simulink library "Lib_NM_NewtonRaphsonSolver_TMATS"  (Simulink 8.5)
settings: Solver=ode45  StartTime=0.0  StopTime=10.0  RelTol=1e-3
Description:
  | Thomas Modules
settings Model: Creator=jwchapm2  LastModifiedBy=jwchapm2

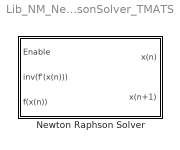
== system Lib_NM_NewtonRaphsonSolver_TMATS ==
  Newton Raphson Solver : Subsystem  TreatAsAtomicUnit=on  mask(T-MATS: Newton Raphson Solver Library Block){NR_IC_M=[1; 2; 3], NR_dx_Lim_M=5, NR_Mx_Lim_M=100000, NR_Mn_Lim_M=0.000001, BlkNm_M=double(gcb)}
      mask prompts: NR_IC_M "NR_IC_M - Initial Conditions of Newton Raphson (mx1)"; NR_dx_Lim_M "NR_dx_Lim_M - Newton Raphson step size limit (%) (1x1)"; NR_Mx_Lim_M "NR_Mx_Lim_M - Max limit (1x1 or mx1)"; NR_Mn_Lim_M "NR_Mn_Lim_M - Min Limit (1x1 or mx1)"; BlkNm_M "BlkNm_M - Block Name"
      mask help:
      | Newton Raphson Solver:
      |
      | x(n+1) = x(n) - inverse(f'(x(n)))*f(x(n))
      |
      | Note:
      | inverse(f'(x(n))) is an m x m matrix and f(x(n)) is an m x 1 matrix
      | where m is the length of the initial conditions matrix and number of system independents.
      mask init:
      | if isequal(size(NR_Mx_Lim_M),size(NR_IC_M))
      | elseif isequal(size(NR_Mx_Lim_M),size(1))
      | else
      |     warning('NR_Mx_Lim_M must be the same size as NR_IC_M or a constant')
      | end
      | 
      | if isequal(size(NR_Mn_Lim_M),size(NR_IC_M))
      | elseif isequal(size(NR_Mn_Lim_M),size(1))
      | else
      |     warning('NR_Mn_Lim_M must be the same size as NR_IC_M or a constant')
      | end
      mask Help: web(which('NumMthd_TMATS_NRS.html'),'-helpbrowser')

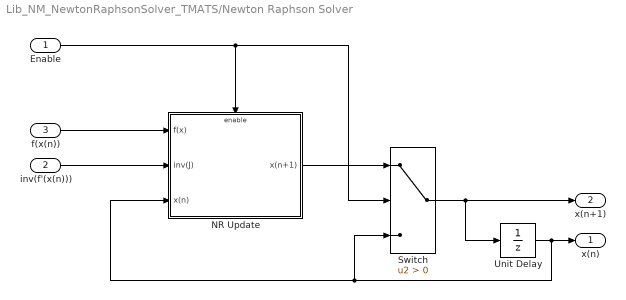
== system Lib_NM_NewtonRaphsonSolver_TMATS/Newton Raphson Solver ==
  Enable : Inport  PortDimensions=1
  inv(f'(x(n))) : Inport  Port=2  PortDimensions=[length(NR_IC_M),length(NR_IC_M)]
  f(x(n)) : Inport  Port=3  PortDimensions=length(NR_IC_M)
  NR Update : Subsystem
  Switch : Switch  Criteria=u2 > Threshold
  Unit Delay : UnitDelay  InitialCondition=NR_IC_M  SampleTime=-1
  x(n) : Outport  PortDimensions=length(NR_IC_M)
  x(n+1) : Outport  Port=2  PortDimensions=length(NR_IC_M)
  wires:
  Unit Delay/1 -> x(n)/1, Switch/3, NR Update/3(x(n))
  Enable/1 -> Switch/2, NR Update/Enable
  Switch/1 -> Unit Delay/1, x(n+1)/1
  f(x(n))/1 -> NR Update/1(f(x))
  inv(f'(x(n)))/1 -> NR Update/2(inv(J))
  NR Update/1(x(n+1)) -> Switch/1

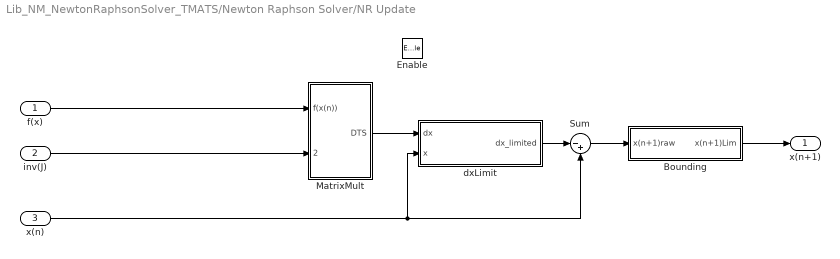
== system Lib_NM_NewtonRaphsonSolver_TMATS/Newton Raphson Solver/NR Update ==
  f(x) : Inport
  inv(J) : Inport  Port=2
  x(n) : Inport  Port=3
  Enable : EnablePort
  Bounding : Subsystem
  MatrixMult : Subsystem
  Sum : Sum  Inputs=|-+
  dxLimit : Subsystem
  x(n+1) : Outport
  wires:
  f(x)/1 -> MatrixMult/1(f(x(n)))
  Sum/1 -> Bounding/1(x(n+1)raw)
  MatrixMult/1(DTS) -> dxLimit/1(dx)
  dxLimit/1(dx_limited) -> Sum/1
  inv(J)/1 -> MatrixMult/2(inv(f'(x(n))))
  Bounding/1(x(n+1)Lim) -> x(n+1)/1
  x(n)/1 -> dxLimit/2(x), Sum/2

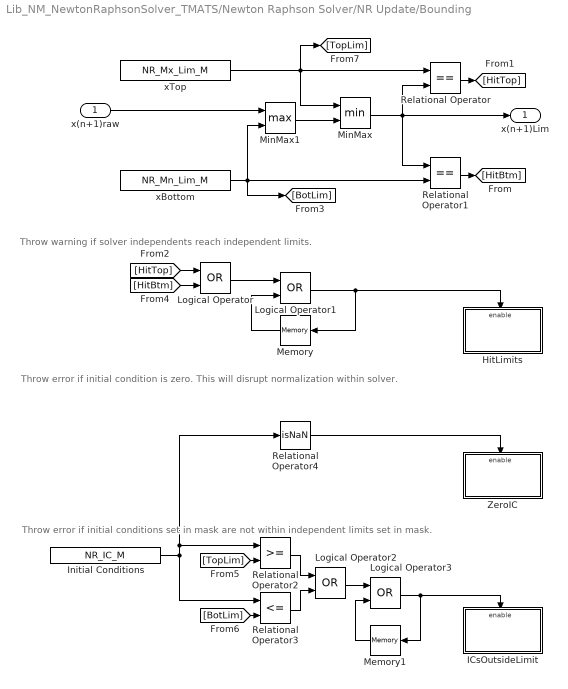
== system Lib_NM_NewtonRaphsonSolver_TMATS/Newton Raphson Solver/NR Update/Bounding ==
  note: Throw error if initial conditions set in mask are not within independent limits set in mask.
  note: Throw error if initial condition is zero. This will disrupt normalization within solver.
  note: Throw warning if solver independents reach independent limits.
  x(n+1)raw : Inport
  HitLimits : Subsystem
  ICsOutsideLimit : Subsystem
  Initial Conditions : Constant  Value=NR_IC_M
  Logical Operator{,1..3} (4 alike) : Logic  Operator=OR  AllPortsSameDT=off  OutDataTypeStr=boolean
  Memory : Memory  InheritSampleTime=on
  Memory1 : Memory  InheritSampleTime=on
  MinMax : MinMax  Inputs=2
  MinMax1 : MinMax  Function=max  Inputs=2
  Relational Operator : RelationalOperator  Operator===  OutDataTypeStr=boolean
  Relational Operator1 : RelationalOperator  Operator===  OutDataTypeStr=boolean
  Relational Operator2 : RelationalOperator  OutDataTypeStr=boolean
  Relational Operator3 : RelationalOperator  Operator=<=  OutDataTypeStr=boolean
  Relational Operator4 : RelationalOperator  Operator=isNaN  OutDataTypeStr=boolean
  ZeroIC : Subsystem
  xBottom : Constant  Value=NR_Mn_Lim_M
  xTop : Constant  Value=NR_Mx_Lim_M
  x(n+1)Lim : Outport
  wires:
  xBottom/1 -> [BotLim], MinMax1/2, Relational Operator1/2
  x(n+1)raw/1 -> MinMax1/1
  xTop/1 -> [TopLim], Relational Operator/1, MinMax/1
  MinMax1/1 -> MinMax/2
  MinMax/1 -> Relational Operator1/1, Relational Operator/2, x(n+1)Lim/1
  Relational Operator1/1 -> [HitBtm]
  Relational Operator/1 -> [HitTop]
  [HitTop] -> Logical Operator/1
  Logical Operator/1 -> Logical Operator1/1
  [HitBtm] -> Logical Operator/2
  Memory/1 -> Logical Operator1/2
  Logical Operator1/1 -> HitLimits/Enable, Memory/1
  Logical Operator3/1 -> ICsOutsideLimit/Enable, Memory1/1
  Initial Conditions/1 -> Relational Operator4/1, Relational Operator2/1, Relational Operator3/1
  [TopLim] -> Relational Operator2/2
  Logical Operator2/1 -> Logical Operator3/1
  Relational Operator3/1 -> Logical Operator2/2
  Memory1/1 -> Logical Operator3/2
  Relational Operator2/1 -> Logical Operator2/1
  [BotLim] -> Relational Operator3/2
  Relational Operator4/1 -> ZeroIC/Enable

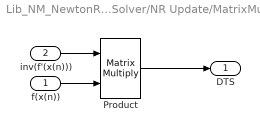
== system Lib_NM_NewtonRaphsonSolver_TMATS/Newton Raphson Solver/NR Update/MatrixMult ==
  f(x(n)) : Inport
  inv(f'(x(n))) : Inport  Port=2
  Product : Product  Multiplication=Matrix(*)  RndMeth=Zero
  DTS : Outport
  wires:
  Product/1 -> DTS/1
  f(x(n))/1 -> Product/2
  inv(f'(x(n)))/1 -> Product/1

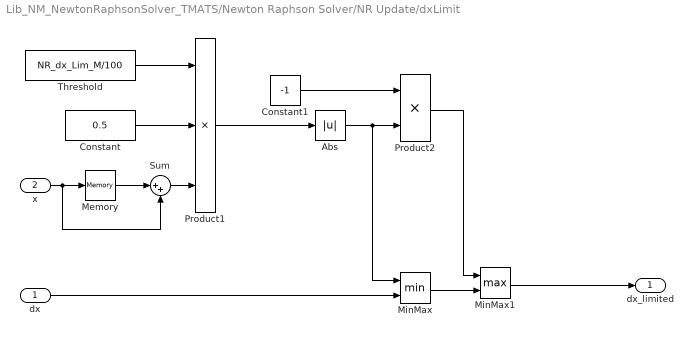
== system Lib_NM_NewtonRaphsonSolver_TMATS/Newton Raphson Solver/NR Update/dxLimit ==
  dx : Inport
  x : Inport  Port=2
  Abs : Abs
  Constant : Constant  Value=0.5
  Constant1 : Constant  Value=-1
  Memory : Memory  X0=NR_IC_M  InheritSampleTime=on
  MinMax : MinMax  Inputs=2
  MinMax1 : MinMax  Function=max  Inputs=2
  Product1 : Product  Inputs=3  RndMeth=Zero
  Product2 : Product  RndMeth=Zero
  Sum : Sum  Inputs=|++
  Threshold : Constant  Value=NR_dx_Lim_M/100
  dx_limited : Outport
  wires:
  MinMax1/1 -> dx_limited/1
  Constant1/1 -> Product2/1
  Product2/1 -> MinMax1/1
  MinMax/1 -> MinMax1/2
  dx/1 -> MinMax/2
  Abs/1 -> Product2/2, MinMax/1
  Product1/1 -> Abs/1
  Threshold/1 -> Product1/1
  x/1 -> Memory/1, Sum/2
  Constant/1 -> Product1/2
  Memory/1 -> Sum/1
  Sum/1 -> Product1/3

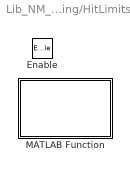
== system Lib_NM_NewtonRaphsonSolver_TMATS/Newton Raphson Solver/NR Update/Bounding/HitLimits ==
  Enable : EnablePort
  MATLAB Function : MATLAB Function  TreatAsAtomicUnit=on

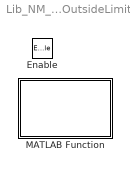
== system Lib_NM_NewtonRaphsonSolver_TMATS/Newton Raphson Solver/NR Update/Bounding/ICsOutsideLimit ==
  Enable : EnablePort
  MATLAB Function : MATLAB Function  TreatAsAtomicUnit=on

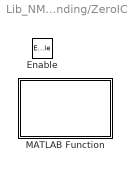
== system Lib_NM_NewtonRaphsonSolver_TMATS/Newton Raphson Solver/NR Update/Bounding/ZeroIC ==
  Enable : EnablePort
  MATLAB Function : MATLAB Function  TreatAsAtomicUnit=on

== matlab function Newton Raphson Solver/NR Update/Bounding/ZeroIC/MATLAB Function ==
  data: BlkNm_M parameter double
function ICIsZero(BlkNm_M)
%# Throw error if initial condition is outside bounds on independent.
BName = BlkNm_M;
error(['Error in ' BName ': Initial conditions, SNR_IC_M, of NR Solver are zero. This will disrupt the normalization within the solver. Please choose non-zero numbers.']);

== matlab function Newton Raphson Solver/NR Update/Bounding/HitLimits/MATLAB Function ==
  data: BlkNm_M parameter double
function fcn(BlkNm_M)
%# Limit Newton Raphson outputs and produce a warning if it occurs
BName = BlkNm_M;
disp(['Warning in ' BName ': Solver limit has been hit, check for system convergence']);

== matlab function Newton Raphson Solver/NR Update/Bounding/ICsOutsideLimit/MATLAB Function ==
  data: BlkNm_M parameter double
function ICNotInsideLimits(BlkNm_M)
%# Throw error if initial condition is outside bounds on independent.
BName = BlkNm_M;
error(['Error in ' BName ': Initial conditions, SNR_IC_M, of NR Solver are not within the Newton Raphson independent limits, SNR_Mx_M and SNR_Mn_M. Please choose initial condiitons conditions within the prescribed limits.']);
